simulink model "LAB1"  (R2018a)
settings: Solver=VariableStepAuto  StartTime=0.0  StopTime=50.0  RelTol=1e-3
libraries: simulink x1
settings Model: Creator=carlos  LastModifiedBy=carlos

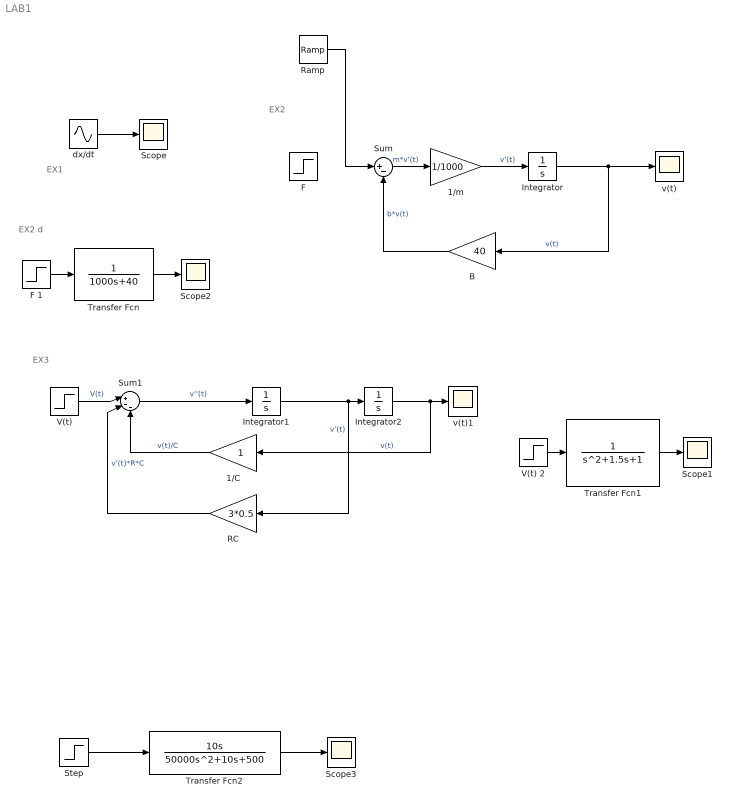
== system LAB1 ==
  note: EX3
  note: EX2
  note: EX1
  note: EX2 d
  1/C : Gain
  1/m : Gain  Gain=1/1000
  "B " : Gain  Gain=40
  "F " : Step  Time=0  After=400  SampleTime=0
  F 1 : Step  Time=0  After=400  SampleTime=0
  Integrator : Integrator
  Integrator1 : Integrator
  Integrator2 : Integrator
  RC : Gain  Gain=3*0.5
  Ramp : simulink/Sources/Ramp  slope=200  start=0  InitialOutput=0
  Scope{,1..3} (4 alike) : Scope
  Step : Step  After=100  SampleTime=0
  Sum : Sum  Inputs=|+-
  Sum1 : Sum  Inputs=|+--
  Transfer Fcn : TransferFcn  Denominator=[1000 40]
  Transfer Fcn1 : TransferFcn  Denominator=[1 1.5 1]
  Transfer Fcn2 : TransferFcn  Numerator=[10 0]  Denominator=[50000 10 500]
  V(t) : Step  Time=0  After=2  SampleTime=0
  V(t) 2 : Step  Time=0  After=2  SampleTime=0
  dx/dt : Sin  Amplitude=3  Frequency=2  SampleTime=0
  v(t) : Scope
  v(t)1 : Scope
  wires:
  dx/dt/1 -> Scope/1
  "B "/1 -> Sum/2  "b*v(t)"
  Sum/1 -> 1/m/1  "m*v'(t)"
  1/m/1 -> Integrator/1  "v'(t)"
  Integrator/1 -> "B "/1, v(t)/1  "v(t)"
  F 1/1 -> Transfer Fcn/1
  Transfer Fcn/1 -> Scope2/1
  Integrator1/1 -> RC/1, Integrator2/1  "v'(t)"
  1/C/1 -> Sum1/3  "v(t)/C"
  Sum1/1 -> Integrator1/1  "v''(t)"
  V(t)/1 -> Sum1/1  "V(t)"
  Integrator2/1 -> 1/C/1, v(t)1/1  "v(t)"
  RC/1 -> Sum1/2  "v'(t)*R*C"
  Transfer Fcn1/1 -> Scope1/1
  V(t) 2/1 -> Transfer Fcn1/1
  Ramp/1 -> Sum/1
  Step/1 -> Transfer Fcn2/1
  Transfer Fcn2/1 -> Scope3/1
